simulink model "OpenLoop_p1"  (R2019b)
settings: Solver=FixedStepAuto  StartTime=0.0  StopTime=10.0  RelTol=1e-3  EnableMultiTasking=on
model workspace (MAT data in the model file):
  P = 36
  TP = 2
undefined symbols (not defined in the file): t_sim
libraries: legoev3lib x6, simulink x1
settings Model: ExtModeTrigDuration=2  Creator=alumnopr18  LastModifiedBy=alumnopr18
settings SolverCC: PositivePriorityOrder=on
settings OptimizationCC: EnhancedBackFolding=on  PassReuseOutputArgsAs=Individual arguments  ZeroExternalMemoryAtStartup=off  ZeroInternalMemoryAtStartup=off  MaxStackSize=64  OptimizeBlockOrder=speed  DifferentSizesBufferReuse=on  OptimizationCustomize=off  EfficientTunableParamExpr=on
settings DebuggingCC: ParameterTunabilityLossMsg=error
settings HardwareCC: ProdBitPerPointer=32  ProdBitPerSizeT=32  ProdBitPerPtrDiffT=32  ProdLargestAtomicInteger=Long  ProdWordSize=32  ProdHWDeviceType=ARM Compatible->ARM 9
settings SFSimCC: MATLABDynamicMemAlloc=off
settings RTWCC: SystemTargetFile=ert.tlc  HardwareBoard=LEGO MINDSTORMS EV3  TLCOptions="-aInlineSetEventsForThisBaseRateFcn=TLC_FALSE -aSuppressMultiTaskScheduler=TLC_FALSE  -aRateBasedStepFcn=0"  TemplateMakefile=ert_default_tmf  GenerateReport=on  Toolchain=Sourcery G++ Lite v2009q3  IncludeHyperlinkInReport=on  LaunchReport=on  GenerateTraceInfo=on  GenerateTraceReport=on  GenerateTraceReportSl=on  GenerateTraceReportSf=on  GenerateTraceReportEml=on
settings CodeAppCC: ForceParamTrailComments=on  IgnoreCustomStorageClasses=off  OperatorAnnotations=on  SimulinkDataObjDesc=on  SFDataObjDesc=on  InsertBlockDesc=on
settings ERTTargetCC: SupportContinuousTime=on  SupportVariableSizeSignals=on

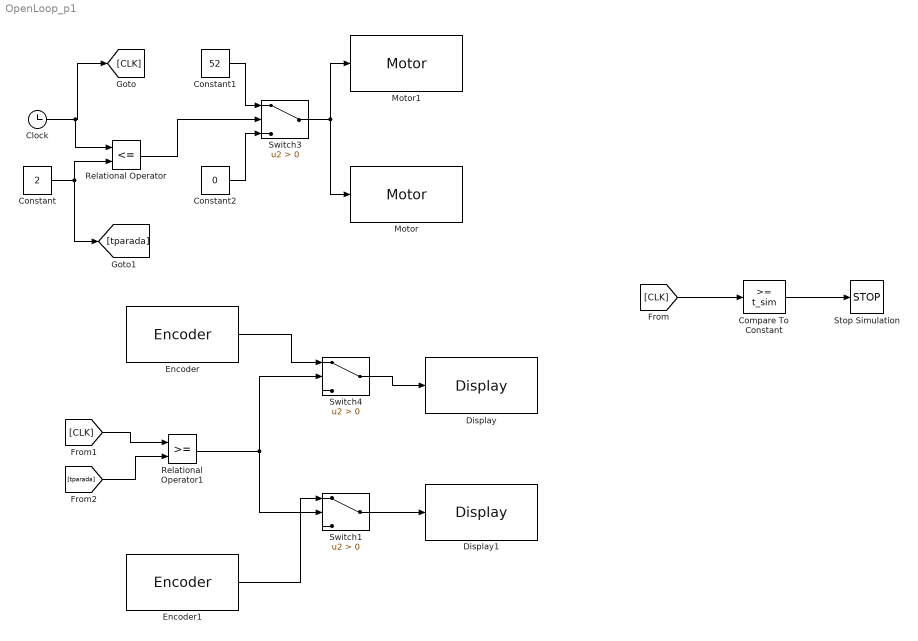
== system OpenLoop_p1 ==
  Clock : Clock
  Compare To Constant : simulink/Logic and Bit Operations/Compare To Constant  relop=>=  const=t_sim  OutDataTypeStr=boolean
  Constant : Constant  Value=2
  Constant1 : Constant  Value=52
  Constant2 : Constant  Value=0
  Display : legoev3lib/Display  slcdLine=1  slcdFormat=Decimal
      settings: SourceProductName=Simulink Support Package for LEGO MINDSTORMS EV3 Hardware  SourceProductBaseCode=LEGOEV3
  Display1 : legoev3lib/Display  slcdLine=2  slcdFormat=Decimal
      settings: SourceProductName=Simulink Support Package for LEGO MINDSTORMS EV3 Hardware  SourceProductBaseCode=LEGOEV3
  Encoder : legoev3lib/Encoder  portNumber=B  opMode=No reset  sampleTime=0.1
      settings: SourceProductName=Simulink Support Package for LEGO MINDSTORMS EV3 Hardware  SourceProductBaseCode=LEGOEV3
  Encoder1 : legoev3lib/Encoder  portNumber=C  opMode=No reset  sampleTime=0.1
      settings: SourceProductName=Simulink Support Package for LEGO MINDSTORMS EV3 Hardware  SourceProductBaseCode=LEGOEV3
  Motor : legoev3lib/Motor  sportNumber=C  sstopAction=Brake
  Motor1 : legoev3lib/Motor  sportNumber=B  sstopAction=Brake
  Relational Operator : RelationalOperator  Operator=<=  OutDataTypeStr=boolean  RndMeth=Simplest
  Relational Operator1 : RelationalOperator  OutDataTypeStr=boolean  RndMeth=Simplest
  Stop Simulation : Stop
  Switch1 : Switch  Criteria=u2 > Threshold
  Switch3 : Switch  Criteria=u2 > Threshold
  Switch4 : Switch  Criteria=u2 > Threshold
  wires:
  Clock/1 -> Relational Operator/1, [CLK]
  [CLK] -> Compare To Constant/1
  Compare To Constant/1 -> Stop Simulation/1
  Constant/1 -> [tparada], Relational Operator/2
  Relational Operator/1 -> Switch3/2
  Constant1/1 -> Switch3/1
  Constant2/1 -> Switch3/3
  Switch3/1 -> Motor/1, Motor1/1
  Switch4/1 -> Display/1
  Switch1/1 -> Display1/1
  [tparada] -> Relational Operator1/2
  [CLK] -> Relational Operator1/1
  Relational Operator1/1 -> Switch1/2, Switch4/2
  Encoder/1 -> Switch4/1
  Encoder1/1 -> Switch1/1
